simulink model "joystick"  (R2022a)
settings: Solver=FixedStepDiscrete  StartTime=0.0  StopTime=inf  FixedStep=0.001  RelTol=1e-3  EnableMultiTasking=on
libraries: slrealtimeutilitieslib x1, vrlib x1, slrealtimeiplib x1
settings Model: Creator=timo.straessle  LastModifiedBy=speedgoat
settings SolverCC: ConcurrentTasks=on  AlgebraicLoopSolver=TrustRegion  PositivePriorityOrder=on  InsertRTBMode=Never (minimum delay)
settings DataIOCC: SaveFormat=Array  SaveState=on  SignalLoggingName=logsOut
settings OptimizationCC: BlockReduction=off  BooleanDataType=off  OptimizeBlockIOStorage=off  BufferReuse=off  GlobalBufferReuse=off  ExpressionFolding=off  LocalBlockOutputs=off  InitFltsAndDblsToZero=on  OptimizeDataStoreBuffers=off  BusAssignmentInplaceUpdate=off
settings DebuggingCC: SaveWithParameterizedLinksMsg=none  UnderspecifiedInitializationDetection=Classic  MergeDetectMultiDrivingBlocksExec=none  CheckExecutionContextPreStartOutputMsg=on  SignalResolutionControl=TryResolveAllWithWarning  TasksWithSamePriorityMsg=none  UnconnectedInputMsg=warning  UnconnectedOutputMsg=warning  UnconnectedLineMsg=warning  SFUnexpectedBacktrackingDiag=warning  SFNoUnconditionalDefaultTransitionDiag=warning  SFExecutionAtInitializationDiag=none  SFMachineParentedDataDiag=warning  ArithmeticOperatorsInVariantConditions=warning
settings HardwareCC: ProdBitPerLong=64  ProdLongLongMode=on  ProdHWDeviceType=Intel->x86-64 (Linux 64)
settings ModelReferenceCC: PropagateSignalLabelsOutOfModel=off
settings SFSimCC: SimUseLocalCustomCode=off  SimTargetLang=C++
settings RTWCC: Description=Simulink Real-Time  SystemTargetFile=slrealtime.tlc  TemplateMakefile=slrealtime_default_tmf  RTWUseLocalCustomCode=off  Toolchain=Simulink Real-Time Toolchain  BuildConfiguration=Faster Runs  CodeExecutionProfiling=on  TargetLang=C++  DLArmComputeVersion=19.05
settings CodeAppCC: StateflowObjectComments=on
settings SimulinkRealTimeTargetCC: MATLABClassNameForMDSCustomization=Simulink.SoftwareTarget.GRTCustomization  UseGCCFastMath=on
settings ConfigComp: CovMetricSettings=dw  CovSaveCumulativeToWorkspaceVar=on  CovSaveSingleToWorkspaceVar=on  CovExternalEMLEnable=off  CovSFcnEnable=off

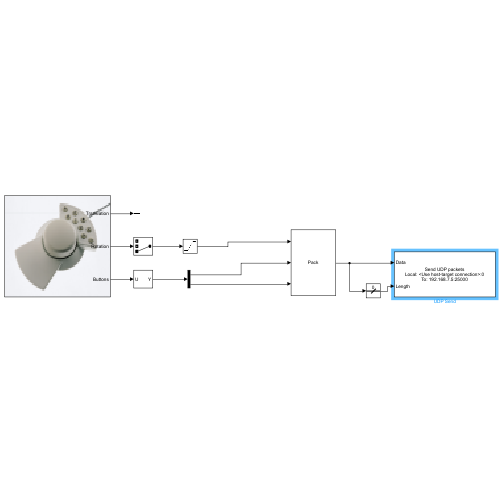
[thumbnail: Simulink's stored preview of the top-level diagram]
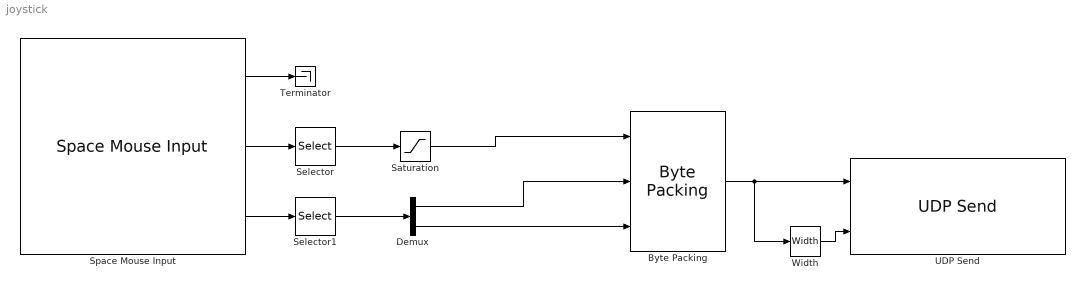
== system joystick ==
  Byte Packing : slrealtimeutilitieslib/Byte Packing  MaskPackedDataType=uint8  MaskUnpackedDataTypes={'double','double','double'}  MaskAlignment=1
  Demux : Demux  Outputs=2
  Saturation : Saturate  UpperLimit=1800  LowerLimit=-1800
  Selector : Selector  InputPortWidth=3  IndexOptions=Index vector (dialog)  Indices=3  OutputSizes=1
  Selector1 : Selector  InputPortWidth=12  IndexOptions=Index vector (dialog)  Indices=[1:2]  OutputSizes=1
  Space Mouse Input : vrlib/Space Mouse Input  Port=USB1  OutputType=Position  Dominant=off  DisableTranslation=off  DisableRotation=off  NormalizeAngle=off  EnableLimit=off  PositionSensitivity=0.0001  RotationSensitivity=0.0001  InitialPosition=[0 0 0]  InitialRotation=[0 0 0]  PositionLow=[-100 -100 -100]  PositionUp=[100 100 100]
      settings: SourceProductBaseCode=SL
  Terminator : Terminator
  UDP Send : slrealtimeiplib/UDP Send  useHostTargetConn=on  toAddress='192.168.7.5'  toPort=25000  sampleTime=-1  enableMessage=off  ipAddress='192.168.7.2'  localPort=-1
      settings: SourceProductBaseCode=XP
  Width : Width
  wires:
  Space Mouse Input/1 -> Terminator/1
  Space Mouse Input/3 -> Selector1/1
  Saturation/1 -> Byte Packing/1
  Byte Packing/1 -> Width/1, UDP Send/1
  Width/1 -> UDP Send/2
  Space Mouse Input/2 -> Selector/1
  Selector/1 -> Saturation/1
  Selector1/1 -> Demux/1
  Demux/1 -> Byte Packing/2
  Demux/2 -> Byte Packing/3
